simulink model "MPC_dlx_control"  (R2022b)
settings: Solver=VariableStepAuto  StartTime=0.0  StopTime=50  RelTol=1e-3
undefined symbols (not defined in the file or in its folder): cx
libraries: Solver_SF x1, simulink x1, slpidlib x1
settings Model: Creator=admin  LastModifiedBy=admin

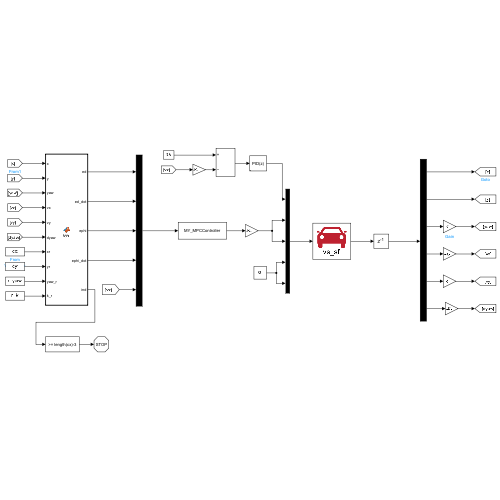
[thumbnail: Simulink's stored preview of the top-level diagram]
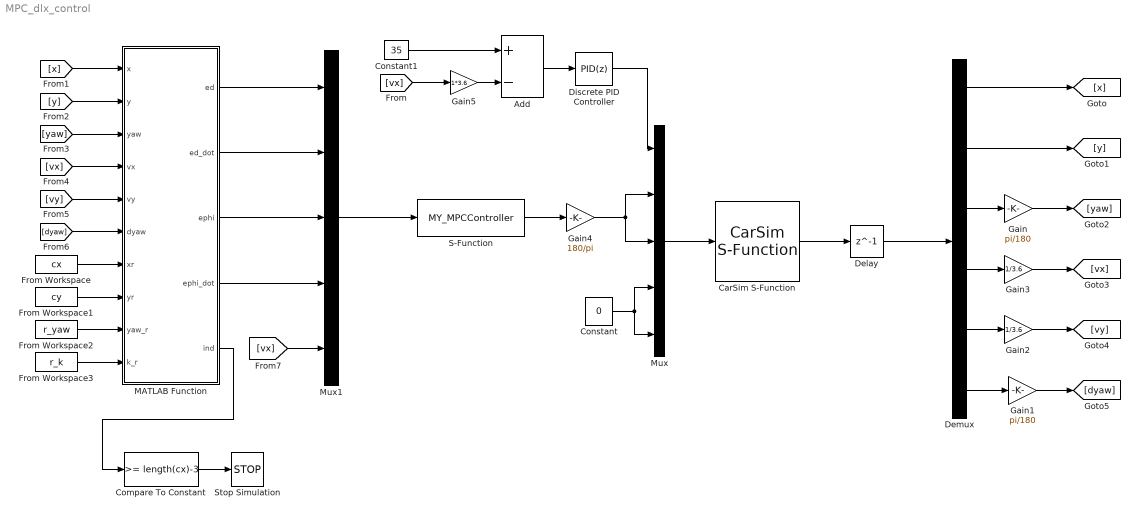
== system MPC_dlx_control ==
  Add : Sum  Inputs=+-
  CarSim S-Function : Solver_SF/CarSim S-Function  Priority=1  SIMFILE=simfile.sim  Run_RTs=off  vs_state_ind=Run  StopMode_ind=Vehicle Model
  Compare To Constant : simulink/Logic and Bit Operations/Compare To Constant  relop=>=  const=length(cx)-3  OutDataTypeStr=boolean
  Constant : Constant  Value=0
  Constant1 : Constant  Value=35
  Delay : Delay  DelayLength=1
  Demux : Demux  Outputs=6
  Discrete PID Controller : slpidlib/PID Controller  Controller=PID  Form=Parallel  TimeDomain=Discrete-time  UseExternalTs=off  SampleTime=-1  IntegratorMethod=Forward Euler  FilterMethod=Forward Euler  ControllerParametersSource=internal  P=0.8  I=0.6  UseKiTs=off  D=0.2  N=100  UseFilter=on  TunerSelectOption=Transfer Function Based (PID Tuner App)  InitialConditionSource=internal  InitialConditionForIntegrator=0  InitialConditionForFilter=0  DifferentiatorICPrevScaledInput=0  ExternalReset=none  TrackingMode=off  Kt=1  LimitOutput=off  SatLimitsSource=internal  UpperSaturationLimit=inf  LowerSaturationLimit=-inf  LinearizeAsGain=off  AntiWindupMode=none  Kb=1  LimitIntegrator=off  UpperIntegratorSaturationLimit=inf  LowerIntegratorSaturationLimit=-inf  POutMin=[]  POutMax=[]  IOutMin=[]  IOutMax=[]  DOutMin=[]  DOutMax=[]  NOutMin=[]  NOutMax=[]  SumOutMin=[]  SumOutMax=[]  SaturationOutMin=[]  SaturationOutMax=[]  PParamMin=[]  PParamMax=[]  IParamMin=[]  IParamMax=[]  DParamMin=[]  DParamMax=[]  NParamMin=[]  NParamMax=[]  KbParamMin=[]  KbParamMax=[]  KtParamMin=[]  KtParamMax=[]  KbOutMin=[]  KbOutMax=[]  KtOutMin=[]  KtOutMax=[]  IntegratorOutMin=[]  IntegratorOutMax=[]  FilterOutMin=[]  FilterOutMax=[]  SumI1OutMin=[]  SumI1OutMax=[]  SumI2OutMin=[]  SumI2OutMax=[]  SumI3OutMin=[]  SumI3OutMax=[]  SumI4OutMin=[]  SumI4OutMax=[]  SumDOutMin=[]  SumDOutMax=[]  DifferentiatorOutMin=[]  DifferentiatorOutMax=[]  FilterDiffOutCoefMin=[]  FilterDiffOutCoefMax=[]  ReciprocalOutMin=[]  ReciprocalOutMax=[]  SumDenOutMin=[]  SumDenOutMax=[]  SumNumOutMin=[]  SumNumOutMax=[]  DivideOutMin=[]  DivideOutMax=[]  UdiffTsProdOutMin=[]  UdiffTsProdOutMax=[]  NTsProdOutMin=[]  NTsProdOutMax=[]  UintegralTsProdOutMin=[]  UintegralTsProdOutMax=[]  UngainTsProdOutMin=[]  UngainTsProdOutMax=[]  ClampingZeroOutDataTypeStr=Inherit: Inherit via back propagation  ClampingZeroOutMin=[]  ClampingZeroOutMax=[]  FilterDenConstantOutDataTypeStr=Inherit: Inherit via back propagation  FilterDenConstantOutMin=[]  FilterDenConstantOutMax=[]  PCopyOutDataTypeStr=Inherit: Inherit via back propagation  PCopyOutMin=[]  PCopyOutMax=[]  NCopyOutDataTypeStr=Inherit: Inherit via back propagation  NCopyOutMin=[]  NCopyOutMax=[]  IntegratorContinuousStateAttributes=''  IntegratorStateMustResolveToSignalObject=off  IntegratorRTWStateStorageClass=Auto  FilterContinuousStateAttributes=''  FilterStateMustResolveToSignalObject=off  FilterRTWStateStorageClass=Auto  ParallelPVariant=InternalParameters  IdealPVariant=Disabled  IVariant=InternalParameters  DVariant=InternalParameters  IntegratorVariant=Discrete  SatVariant=Disabled  AWVariant=Passthrough  PCopyVariant=Disabled  TRVariant=Disabled  FdbkBlocksVariant=Forward  IdealPFdbkVariant=Disabled  SatFdbkVariant=Disabled  DerivativeFilterVariant=ForwardEulerFilter  NVariant=InternalParameters  NCopyVariant=Disabled  FilterICVariant=InternalICsFilter  IntegratorICVariant=InternalICs  ExternalResetVariant=Disabled  TRSumVariant=Passthrough  SumFdbkVariant=Disabled  SumVariant=Sum_PID  TsampFilterVariant=InternalTs  TsampNgainVariant=Passthrough  TsampIntegralVariant=Passthrough  ExternalSaturationOutDataTypeStr=Inherit: Same as second input
      settings: LibrarySourceBlock=simulink/Discrete/Discrete PID Controller
  From Workspace : FromWorkspace  VariableName=cx
  From Workspace1 : FromWorkspace  VariableName=cy
  From Workspace2 : FromWorkspace  VariableName=r_yaw
  From Workspace3 : FromWorkspace  VariableName=r_k
  Gain : Gain  Gain=pi/180
  Gain1 : Gain  Gain=pi/180
  Gain2 : Gain  Gain=1/3.6
  Gain3 : Gain  Gain=1/3.6
  Gain4 : Gain  Gain=180/pi
  Gain5 : Gain  Gain=1*3.6
  MATLAB Function : MATLAB Function  TreatAsAtomicUnit=on
  Mux : Mux  Inputs=5
  Mux1 : Mux  Inputs=5
  S-Function : S-Function  FunctionName=MY_MPCController  SFunctionDeploymentMode=off  EnableBusSupport=off
  Stop Simulation : Stop
  wires:
  CarSim S-Function/1 -> Delay/1
  Delay/1 -> Demux/1
  Demux/3 -> Gain/1
  Gain/1 -> [yaw]
  Demux/6 -> Gain1/1
  Gain1/1 -> [dyaw]
  Demux/5 -> Gain2/1
  Gain2/1 -> [vy]
  Demux/4 -> Gain3/1
  Gain3/1 -> [vx]
  Demux/1 -> [x]
  Demux/2 -> [y]
  Mux/1 -> CarSim S-Function/1
  Constant/1 -> Mux/5, Mux/4
  Gain4/1 -> Mux/3, Mux/2
  [vx] -> Gain5/1
  Gain5/1 -> Add/2
  Constant1/1 -> Add/1
  Add/1 -> Discrete PID Controller/1
  Discrete PID Controller/1 -> Mux/1
  S-Function/1 -> Gain4/1
  MATLAB Function/1(ed) -> Mux1/1
  MATLAB Function/3(ephi) -> Mux1/3
  MATLAB Function/4(ephi_dot) -> Mux1/4
  MATLAB Function/5(ind) -> Compare To Constant/1
  MATLAB Function/2(ed_dot) -> Mux1/2
  [x] -> MATLAB Function/1(x)
  From Workspace/1 -> MATLAB Function/7(xr)
  From Workspace1/1 -> MATLAB Function/8(yr)
  From Workspace3/1 -> MATLAB Function/10(k_r)
  From Workspace2/1 -> MATLAB Function/9(yaw_r)
  [dyaw] -> MATLAB Function/6(dyaw)
  [vy] -> MATLAB Function/5(vy)
  [vx] -> MATLAB Function/4(vx)
  [yaw] -> MATLAB Function/3(yaw)
  [y] -> MATLAB Function/2(y)
  Mux1/1 -> S-Function/1
  [vx] -> Mux1/5
  Compare To Constant/1 -> Stop Simulation/1

== matlab function MPC_dlx_control/MATLAB Function ==
  data: x input; ed output; y input; yaw input; vx input; vy input; dyaw input; xr input; yr input; yaw_r input; k_r input; ed_dot output; ephi output; ephi_dot output; ind output
function [ed,ed_dot,ephi,ephi_dot,ind] = fcn(x,y,yaw, vx,vy,dyaw,xr,yr,yaw_r,k_r)
%1.寻找匹配点（车辆离期望路径最近的点）   
    n=length(xr);
    d_min=(x-xr(1))^2+(y-yr(1))^2;
    min=1;
    for i=1:n
        d=(x-xr(i))^2+(y-yr(i))^2;
        if d<d_min
            d_min=d;
            min=i;
        end
    end
    ind=min;
%2.计算4个误差状态[ed,d_ed,eyaw,d_eyaw]
    tor=[cos(yaw_r(ind));sin(yaw_r(ind))];
    nor=[-sin(yaw_r(ind));cos(yaw_r(ind))];
    d_err=[x-xr(ind);y-yr(ind)];

    ed=nor'*d_err;
%     es=tor'*d_err; 
    projection_point_thetar=yaw_r(ind); %百度apollo

    ed_dot=vy*cos(yaw-projection_point_thetar)+vx*sin(yaw-projection_point_thetar);
    ephi=sin(yaw-projection_point_thetar);
    s_dot=vx*cos(yaw-projection_point_thetar)-vy*sin(yaw-projection_point_thetar);
    s_dot=s_dot/(1-k_r(ind)*ed);
    ephi_dot=dyaw-k_r(ind)*s_dot;

end
